simulink library "buildSqrdExpCovMat_ul"  (R2018b)
settings: Solver=VariableStepAuto  StartTime=0.0  StopTime=10.0  RelTol=1e-3
libraries: calcSqredExpCov_ul x1
settings Model: Creator=asiddiq2  LastModifiedBy=Ayaz

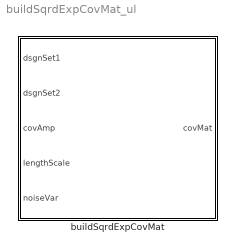
== system buildSqrdExpCovMat_ul ==
  buildSqrdExpCovMat : Subsystem  TreatAsAtomicUnit=on

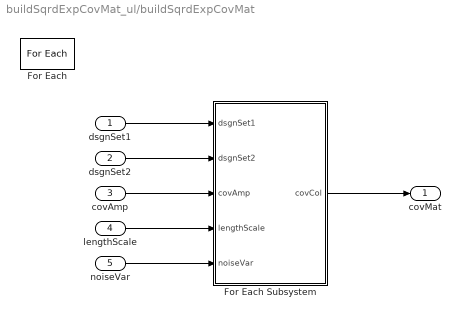
== system buildSqrdExpCovMat_ul/buildSqrdExpCovMat ==
  dsgnSet1 : Inport  Partition=on  PartitionDimension=2  PartitionWidth=1  PartitionOffset=0
  dsgnSet2 : Inport  Port=2
  covAmp : Inport  Port=3
  lengthScale : Inport  Port=4
  noiseVar : Inport  Port=5
  For Each : ForEach  DisableCoverage=on  IndexMode=One-based
  For Each Subsystem : Subsystem  TreatAsAtomicUnit=on
  covMat : Outport  ConcatenationDimension=1
  wires:
  dsgnSet1/1 -> For Each Subsystem/1(dsgnSet1)
  dsgnSet2/1 -> For Each Subsystem/2(dsgnSet2)
  covAmp/1 -> For Each Subsystem/3(covAmp)
  lengthScale/1 -> For Each Subsystem/4(lengthScale)
  For Each Subsystem/1(covCol) -> covMat/1
  noiseVar/1 -> For Each Subsystem/5(noiseVar)

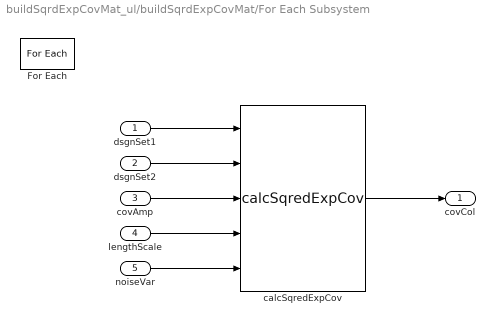
== system buildSqrdExpCovMat_ul/buildSqrdExpCovMat/For Each Subsystem ==
  dsgnSet1 : Inport
  dsgnSet2 : Inport  Port=2  Partition=on  PartitionDimension=2  PartitionWidth=1  PartitionOffset=0
  covAmp : Inport  Port=3
  lengthScale : Inport  Port=4
  noiseVar : Inport  Port=5
  For Each : ForEach  DisableCoverage=on  IndexMode=One-based
  calcSqredExpCov : calcSqredExpCov_ul/calcSqredExpCov  SystemSampleTime=-1
  covCol : Outport  ConcatenationDimension=2
  wires:
  dsgnSet1/1 -> calcSqredExpCov/1
  dsgnSet2/1 -> calcSqredExpCov/2
  covAmp/1 -> calcSqredExpCov/3
  lengthScale/1 -> calcSqredExpCov/4
  calcSqredExpCov/1 -> covCol/1
  noiseVar/1 -> calcSqredExpCov/5
